simulink model "pendulum2D_nonlinear_control_simulation"  (R2017a)
settings: Solver=FixedStepAuto  StartTime=0.0  StopTime=20  FixedStep=dt  RelTol=1e-3
values from neighbouring files (symbols this model uses):
  d = 5    [initialize_controller_pendulum2d_nonlinear.m]    (also in swingCompensator2D.m)
  dt = 1e-3    (= 0.001)    [f_simulink.m]    (also in initialize_controller_pendulum2d_nonlinear.m)
  theta_init = 00*pi/180    (= 0)    [initialize_controller_pendulum2d_nonlinear.m]
  x_init = 0    [initialize_controller_pendulum2d_nonlinear.m]
undefined symbols (not defined in the file or in its folder): KI
libraries: sharedTrackingLibrary x1, simulink x1
settings Model: Creator=Jan  LastModifiedBy=Jan

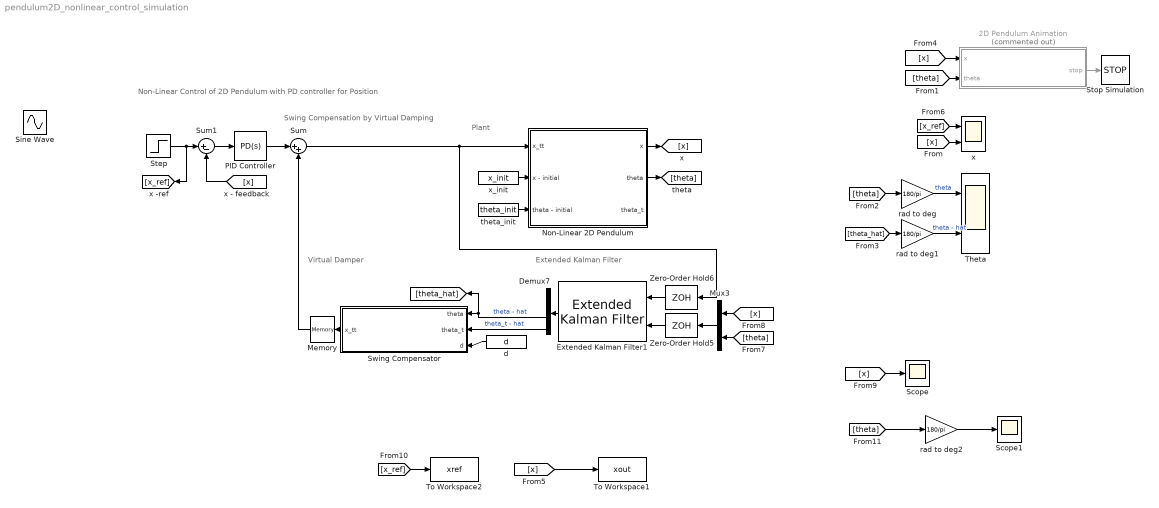
== system pendulum2D_nonlinear_control_simulation ==
  note: Virtual Damper
  note: Plant
  note: Non-Linear Control of 2D Pendulum with PD controller for Position
  note: Swing Compensation by Virtual Damping
  note: Extended Kalman Filter
  2D Pendulum Animation : MATLAB Function  Commented=on  TreatAsAtomicUnit=on  SystemSampleTime=0.1
  Demux7 : Demux
  Extended Kalman Filter1 : sharedTrackingLibrary/Extended Kalman Filter  StateTransitionFcn=f_simulink  HasStateTransitionJacobianFcn=off  HasAdditiveProcessNoise=Additive  ProcessNoise=Q  HasTimeVaryingProcessNoise=off  HasStateTransitionFcnExtraArgument=1  InitialState=x0  InitialStateCovariance=P  MeasurementFcn1=h_simulink  HasMeasurementJacobianFcn1=off  HasMeasurementEnablePort1=off  HasAdditiveMeasurementNoise1=Additive  MeasurementNoise1=R  HasTimeVaryingMeasurementNoise1=off  HasMeasurementFcnExtraArgument1=0  MeasurementFcn2=myMeasurementFcn  HasMeasurementJacobianFcn2=off  HasMeasurementEnablePort2=off  HasAdditiveMeasurementNoise2=Additive  MeasurementNoise2=1  HasTimeVaryingMeasurementNoise2=off  HasMeasurementFcnExtraArgument2=0  MeasurementFcn3=myMeasurementFcn  HasMeasurementJacobianFcn3=off  HasMeasurementEnablePort3=off  HasAdditiveMeasurementNoise3=Additive  MeasurementNoise3=1  HasTimeVaryingMeasurementNoise3=off  HasMeasurementFcnExtraArgument3=0  MeasurementFcn4=myMeasurementFcn  HasMeasurementJacobianFcn4=off  HasMeasurementEnablePort4=off  HasAdditiveMeasurementNoise4=Additive  MeasurementNoise4=1  HasTimeVaryingMeasurementNoise4=off  HasMeasurementFcnExtraArgument4=0  MeasurementFcn5=myMeasurementFcn  HasMeasurementJacobianFcn5=off  HasMeasurementEnablePort5=off  HasAdditiveMeasurementNoise5=Additive  MeasurementNoise5=1  HasTimeVaryingMeasurementNoise5=off  HasMeasurementFcnExtraArgument5=0  EnableMultirate=off  StateTransitionFcnSampleTime=1  MeasurementFcn1SampleTime=1  MeasurementFcn2SampleTime=1  MeasurementFcn3SampleTime=1  MeasurementFcn4SampleTime=1  MeasurementFcn5SampleTime=1  UseCurrentEstimator=on  OutputStateCovariance=off  DataType=double  SampleTime=dt  NumberOfMeasurements=1
  Memory : Memory
  Mux3 : Mux  Inputs=2
  Non-Linear 2D Pendulum : Subsystem
  PID Controller : simulink/Continuous/PID Controller  Controller=PD  TimeDomain=Continuous-time  SampleTime=-1  IntegratorMethod=Forward Euler  FilterMethod=Forward Euler  Form=Parallel  UseFilter=on  ControllerParametersSource=internal  P=0.2  I=KI  D=0.85  N=100  InitialConditionSource=internal  InitialConditionForIntegrator=0  InitialConditionForFilter=0  ExternalReset=none  LimitOutput=off  UpperSaturationLimit=inf  LowerSaturationLimit=-inf  LinearizeAsGain=on  AntiWindupMode=none  Kb=1  TrackingMode=off  Kt=1  PParamMin=[]  PParamMax=[]  IParamMin=[]  IParamMax=[]  DParamMin=[]  DParamMax=[]  NParamMin=[]  NParamMax=[]  KbParamMin=[]  KbParamMax=[]  KtParamMin=[]  KtParamMax=[]  POutMin=[]  POutMax=[]  IOutMin=[]  IOutMax=[]  DOutMin=[]  DOutMax=[]  NOutMin=[]  NOutMax=[]  KbOutMin=[]  KbOutMax=[]  KtOutMin=[]  KtOutMax=[]  IntegratorOutMin=[]  IntegratorOutMax=[]  FilterOutMin=[]  FilterOutMax=[]  SumOutMin=[]  SumOutMax=[]  SumI1OutMin=[]  SumI1OutMax=[]  SumI2OutMin=[]  SumI2OutMax=[]  SumI3OutMin=[]  SumI3OutMax=[]  SumDOutMin=[]  SumDOutMax=[]  SaturationOutMin=[]  SaturationOutMax=[]  IntegratorContinuousStateAttributes=''  IntegratorStateMustResolveToSignalObject=off  IntegratorRTWStateStorageClass=Auto  FilterContinuousStateAttributes=''  FilterStateMustResolveToSignalObject=off  FilterRTWStateStorageClass=Auto  DifferentiatorICPrevScaledInput=0  DifferentiatorOutMin=[]  DifferentiatorOutMax=[]  InitialConditionSetting=State (most efficient)
  Scope : Scope
  Scope1 : Scope
  Sine Wave : Sin  Frequency=2*pi*0.1  SampleTime=0
  Step : Step  Time=0  SampleTime=0
  Stop Simulation : Stop
  Sum : Sum  Inputs=|++
  Sum1 : Sum  Inputs=|+-
  Swing Compensator : MATLAB Function  TreatAsAtomicUnit=on
  Theta : Scope  NumInputPorts=2
  To Workspace1 : ToWorkspace  VariableName=xout  SampleTime=-1
  To Workspace2 : ToWorkspace  VariableName=xref  SampleTime=-1
  Zero-Order Hold5 : ZeroOrderHold  SampleTime=dt
  Zero-Order Hold6 : ZeroOrderHold  SampleTime=dt
  d : Constant  Value=d
  rad to deg : Gain  Gain=180/pi
  rad to deg1 : Gain  Gain=180/pi
  rad to deg2 : Gain  Gain=180/pi
  theta_init : Constant  Value=theta_init
  x : Scope  NumInputPorts=2
  x_init : Constant  Value=x_init
  wires:
  Non-Linear 2D Pendulum/2(theta) -> [theta]
  Sum/1 -> Zero-Order Hold6/1, Non-Linear 2D Pendulum/1(x_tt)
  Demux7/4 -> Swing Compensator/2(theta_t)  "theta_t - hat"
  x_init/1 -> Non-Linear 2D Pendulum/2(x - initial)
  d/1 -> Swing Compensator/3(d)
  Swing Compensator/1(x_tt) -> Memory/1
  Memory/1 -> Sum/2
  Sum1/1 -> PID Controller/1
  rad to deg/1 -> Theta/1  "theta"
  [theta] -> rad to deg/1
  rad to deg1/1 -> Theta/2  "theta - hat"
  [theta_hat] -> rad to deg1/1
  [x_ref] -> x/1
  [x] -> Mux3/1
  Zero-Order Hold5/1 -> Extended Kalman Filter1/2
  Extended Kalman Filter1/1 -> Demux7/1
  [theta] -> Mux3/2
  Zero-Order Hold6/1 -> Extended Kalman Filter1/1
  Mux3/1 -> Zero-Order Hold5/1
  Non-Linear 2D Pendulum/1(x) -> [x]
  theta_init/1 -> Non-Linear 2D Pendulum/3(theta - initial)
  Demux7/3 -> [theta_hat], Swing Compensator/1(theta)  "theta - hat"
  [x] -> x/2
  [x] -> 2D Pendulum Animation/1(x)
  2D Pendulum Animation/1(stop) -> Stop Simulation/1
  [theta] -> 2D Pendulum Animation/2(theta)
  [x] -> Sum1/2
  [x] -> To Workspace1/1
  [x_ref] -> To Workspace2/1
  Step/1 -> [x_ref], Sum1/1
  PID Controller/1 -> Sum/1
  [x] -> Scope/1
  rad to deg2/1 -> Scope1/1
  [theta] -> rad to deg2/1

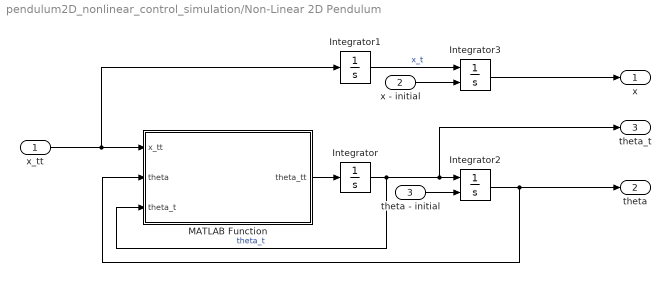
== system pendulum2D_nonlinear_control_simulation/Non-Linear 2D Pendulum ==
  x_tt : Inport
  x - initial : Inport  Port=2
  theta - initial : Inport  Port=3
  Integrator : Integrator
  Integrator1 : Integrator
  Integrator2 : Integrator  InitialConditionSource=external
  Integrator3 : Integrator  InitialConditionSource=external
  MATLAB Function : MATLAB Function  TreatAsAtomicUnit=on
  x : Outport
  theta : Outport  Port=2
  theta_t : Outport  Port=3
  wires:
  Integrator/1 -> MATLAB Function/3(theta_t), Integrator2/1, theta_t/1  "theta_t"
  x_tt/1 -> MATLAB Function/1(x_tt), Integrator1/1
  x - initial/1 -> Integrator3/2
  Integrator1/1 -> Integrator3/1  "x_t"
  MATLAB Function/1(theta_tt) -> Integrator/1
  theta - initial/1 -> Integrator2/2
  Integrator2/1 -> MATLAB Function/2(theta), theta/1
  Integrator3/1 -> x/1

== matlab function pendulum2D_nonlinear_control_simulation/Non-Linear 2D Pendulum/MATLAB Function ==
  data: x_tt input; theta input; theta_tt output; theta_t input
function theta_tt = pendulum_dynamics(x_tt, theta, theta_t)
    
    % Constants
    g = 9.81;   % Gravity
    L = 2.0;    % Wire length
    
    % Pendulum ODE
    theta_tt = (-g*sin(theta) - cos(theta)*x_tt)/L;

== matlab function pendulum2D_nonlinear_control_simulation/Swing Compensator ==
  data: theta input; x_tt output; theta_t input; d input
function x_tt = swingCompensator2D(theta, theta_t, d)
    % Compute the virtual damping to the simple pendulum system
    
    % Constants
    g = 9.81;   % Gravity [m/s^2]
    L = 2.0;    % Wire length
    x_tt = d*L*theta_t/cos(theta);
end

== matlab function pendulum2D_nonlinear_control_simulation/2D Pendulum Animation ==
  data: x input; stop output; theta input
function stop = SimulinkPendulumPlot(x, theta)
    % Creates a 2D-animation for the pendulum motion
    % Input:
    %   xt :   Position of tool-point
    %   theta : Euler angle of pendulum
    % Output:
    %   stop : Bool value to stop the animation
    
    % Persistent variables, to only be initialized once
    persistent h;           % Plot
    persistent L;
    
    stop = false;
    
    %% Initialization 
    % One time intitialization of plotting settings
    if isempty(h)
        % Plotting setup
        h = figure('Name','StewartPlatform Animation');
        L = 2.0;
        xlabel('x-axis')
        ylabel('y-axis')
%         zlabel('z-axis')
        xlim([-5, 5])
        ylim([-5, 1])
%         zlim([0, 8])
        hold on;
        grid on;
%         view(-40,20);
    end
    
     %% Drawing
    if ishandle(h)
        cla;
        Pt = [x, 0];
        Pp = Pt + L*[sin(theta), -cos(theta)];
        
        plot_line(Pt, Pp);
        plot(Pp(1), Pp(2), 'ro', 'LineWidth', 2);

        drawnow;
    end
    
    %% Destructor
    if ~ishandle(h)
        stop = true;
    end

    function plot_line(p1, p2)
%         Pre-allocate
        line = zeros(2,2);
        line(1,:) = p1;
        line(2,:) = p2;

        plot(line(:,1), line(:,2), 'k')
    end
end
